simulink model "MyModel"  (R2024b)
settings: Solver=VariableStepAuto  StartTime=0.0  StopTime=20  RelTol=1e-3
undefined symbols (not defined in the file): Ad, Bd, Cd, d1, d2, g, g_q, K_d, L, mc, mp, Ob, Ts, x0

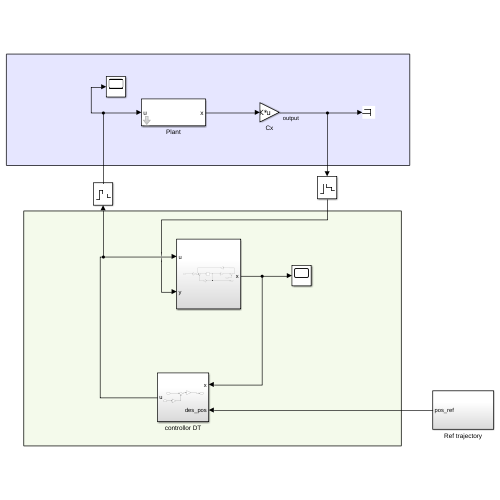
[thumbnail: Simulink's stored preview of the top-level diagram]
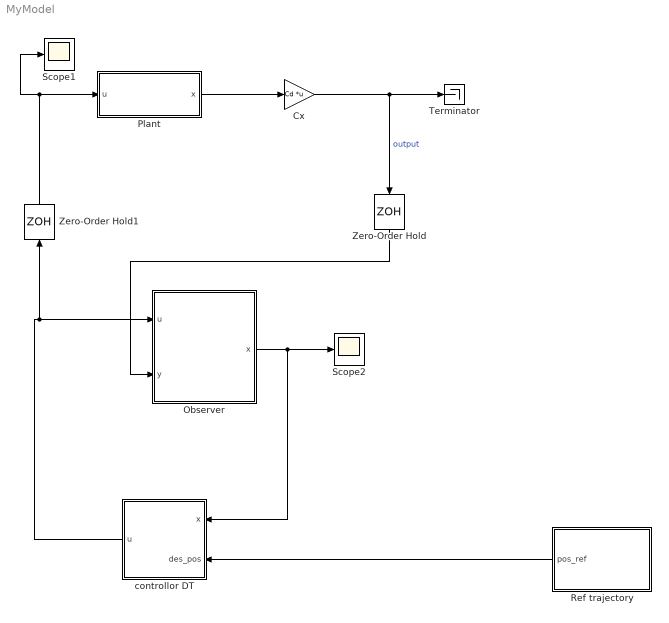
== system MyModel ==
  Cx : Gain  Gain=Cd  Multiplication=Matrix(K*u)
  Observer : Subsystem
  Plant : Subsystem  mask{mp=mp, mc=mc, L=L, g=g, g_q=g_q, d1=d1, d2=d2, x_0=x0}
      mask help:
      | ---------------------------
      | TU Kaiserslautern, LRS
      | Ali Turnwald
      | Last Edit: 19.11.2015
      | ---------------------------
      |
      |
      | A non-linear model for the cart-pendulum system for simulation and animation
      |
      | mc = Mass of the cart
      | mp = Mass of the pendulum
      | g =  Earth gravity
      | L =  Length of the pendulum
      | d1 = Damping of the cart displacement
      | d2 = Damping in the joint
      | x_0 = The vector af initail state [4x1]
      mask DialogControl Text Prompt: Cart-Pendulum System
      mask Display:
      | port_label('output', 1, 'x')
      | port_label('input', 1, 'u')
  Ref trajectory : Subsystem
  Scope1 : Scope
  Scope2 : Scope
  Terminator : Terminator
  Zero-Order Hold : ZeroOrderHold  SampleTime=Ts
  Zero-Order Hold1 : ZeroOrderHold  SampleTime=Ts
  controllor DT : Subsystem
  wires:
  controllor DT/1(u) -> Observer/1(u), Zero-Order Hold1/1
  Ref trajectory/1(pos_ref) -> controllor DT/2(des_pos)
  Zero-Order Hold1/1 -> Plant/1(u), Scope1/1
  Zero-Order Hold/1 -> Observer/2(y)
  Observer/1(x) -> controllor DT/1(x), Scope2/1
  Plant/1(x) -> Cx/1
  Cx/1 -> Terminator/1, Zero-Order Hold/1  "output"

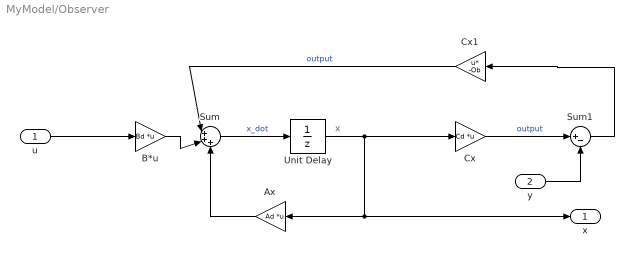
== system MyModel/Observer ==
  note: x
  u : Inport
  y : Inport  Port=2
  Ax : Gain  Gain=Ad  Multiplication=Matrix(K*u) (u vector)
  B*u : Gain  Gain=Bd  Multiplication=Matrix(K*u)
  Cx : Gain  Gain=Cd  Multiplication=Matrix(K*u)
  Cx1 : Gain  Gain=-Ob  Multiplication=Matrix(u*K)
  Sum : Sum  Inputs=|+++
  Sum1 : Sum  Inputs=|+-
  Unit Delay : UnitDelay  SampleTime=-1  HasFrameUpgradeWarning=on
  x : Outport
  wires:
  Sum/1 -> Unit Delay/1  "x_dot"
  u/1 -> B*u/1
  Ax/1 -> Sum/3
  Unit Delay/1 -> x/1, Ax/1, Cx/1
  Cx/1 -> Sum1/1  "output"
  y/1 -> Sum1/2
  Sum1/1 -> Cx1/1
  B*u/1 -> Sum/2
  Cx1/1 -> Sum/1  "output"

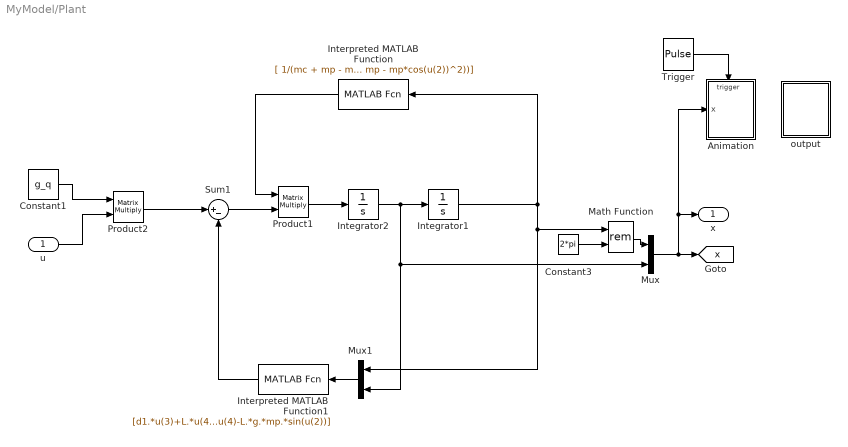
== system MyModel/Plant ==
  u : Inport
  Animation : Subsystem
  Constant1 : Constant  Value=g_q
  Constant3 : Constant  Value=2*pi
  Integrator1 : Integrator  InitialCondition=x_0(1:2)
  Integrator2 : Integrator  InitialCondition=x_0(3:4)
  Interpreted MATLAB Function : MATLABFcn  MATLABFcn="[ 1/(mc + mp - mp*cos(u(2))^2),        cos(u(2))/(L*(mc + mp - mp*cos(u(2))^2)); cos(u(2))/(L*(mc + mp - mp*cos(u(2))^2)), (mc + mp)/(L^2*mp*(mc + mp - mp*cos(u(2))^2))]"  Output1D=off
  Interpreted MATLAB Function1 : MATLABFcn  MATLABFcn=[d1.*u(3)+L.*u(4).^2.*mp.*sin(u(2));d2.*u(4)-L.*g.*mp.*sin(u(2))]
  Math Function : Math  Operator=rem  SignedPower=on
  Mux : Mux  Inputs=2
  Mux1 : Mux  Inputs=2
  Product1 : Product  Multiplication=Matrix(*)
  Product2 : Product  Multiplication=Matrix(*)
  Sum1 : Sum  Inputs=|+-
  Trigger : DiscretePulseGenerator  PulseType=Time based  Period=0.1  PulseWidth=50
  output : Subsystem
  x : Outport  VectorParamsAs1DForOutWhenUnconnected=off
  tag scope: x=global
  wires:
  Integrator2/1 -> Mux1/2, Mux/2, Integrator1/1
  Product1/1 -> Integrator2/1
  Integrator1/1 -> Interpreted MATLAB Function/1, Mux1/1, Math Function/1
  Interpreted MATLAB Function/1 -> Product1/1
  Sum1/1 -> Product1/2
  Interpreted MATLAB Function1/1 -> Sum1/2
  Constant1/1 -> Product2/1
  u/1 -> Product2/2
  Mux/1 -> Animation/1(x), x/1, [x]
  Math Function/1 -> Mux/1
  Constant3/1 -> Math Function/2
  Product2/1 -> Sum1/1
  Trigger/1 -> Animation/Trigger
  Mux1/1 -> Interpreted MATLAB Function1/1

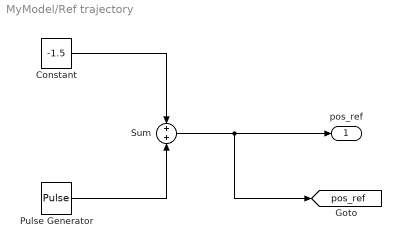
== system MyModel/Ref trajectory ==
  Constant : Constant  Value=-1.5
  Pulse Generator : DiscretePulseGenerator  PulseType=Time based  Amplitude=3  Period=20  PulseWidth=50
  Sum : Sum
  pos_ref : Outport  VectorParamsAs1DForOutWhenUnconnected=off
  tag scope: pos_ref=global
  wires:
  Sum/1 -> [pos_ref], pos_ref/1
  Pulse Generator/1 -> Sum/2
  Constant/1 -> Sum/1

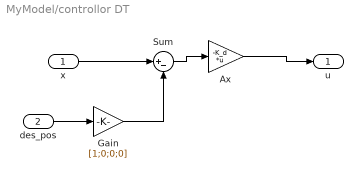
== system MyModel/controllor DT ==
  x : Inport
  des_pos : Inport  Port=2
  Ax : Gain  Gain=-K_d  Multiplication=Matrix(K*u)
  Gain : Gain  Gain=[1;0;0;0]
  Sum : Sum  Inputs=|+-
  u : Outport
  wires:
  Ax/1 -> u/1
  x/1 -> Sum/1
  Sum/1 -> Ax/1
  des_pos/1 -> Gain/1
  Gain/1 -> Sum/2

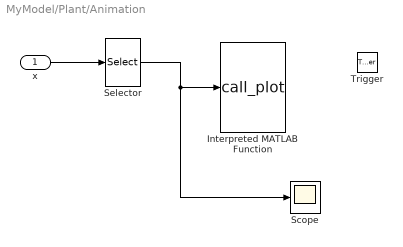
== system MyModel/Plant/Animation ==
  x : Inport
  Trigger : TriggerPort  VariantControl=(inherit)  PortDimensions=1
  Interpreted MATLAB Function : MATLABFcn  MATLABFcn=call_plot  OutputDimensions=0
  Scope : Scope
  Selector : Selector  InputPortWidth=4  IndexOptions=Index vector (dialog)  Indices=[1:2]  OutputSizes=1
  wires:
  x/1 -> Selector/1
  Selector/1 -> Scope/1, Interpreted MATLAB Function/1

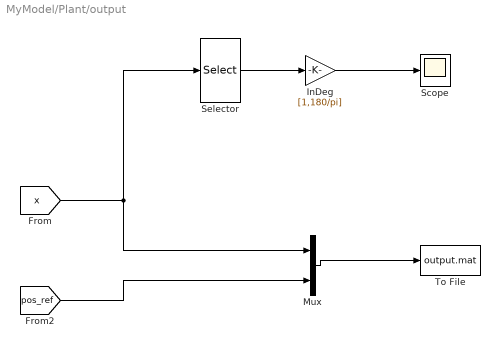
== system MyModel/Plant/output ==
  InDeg : Gain  Gain=[1,180/pi]
  Mux : Mux  Inputs=2
  Scope : Scope
  Selector : Selector  InputPortWidth=4  IndexOptions=Index vector (dialog)  Indices=[1:2]  OutputSizes=1
  To File : ToFile  Filename=output.mat  MatrixName=out  SaveFormat=Timeseries
  wires:
  [x] -> Mux/1, Selector/1
  InDeg/1 -> Scope/1
  Selector/1 -> InDeg/1
  Mux/1 -> To File/1
  [pos_ref] -> Mux/2
